simulink model "bat_cycling"  (R2021b)
settings: Solver=VariableStepAuto  StartTime=0.0  StopTime=3600*8640  RelTol=1e-3
undefined symbols (not defined in the file): Ion, Lithium
libraries: spsBatteryLib x1, spsControlledCurrentSourceLib x1, slpidlib x1, spspowerguiLib x1
settings Model: SimulationMode=accelerator  Creator=anna897  LastModifiedBy=anna897

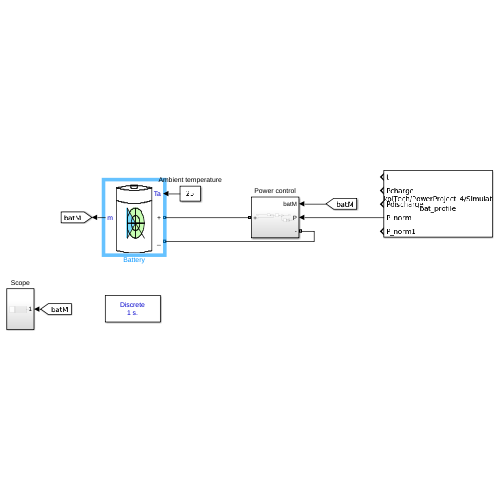
[thumbnail: Simulink's stored preview of the top-level diagram]
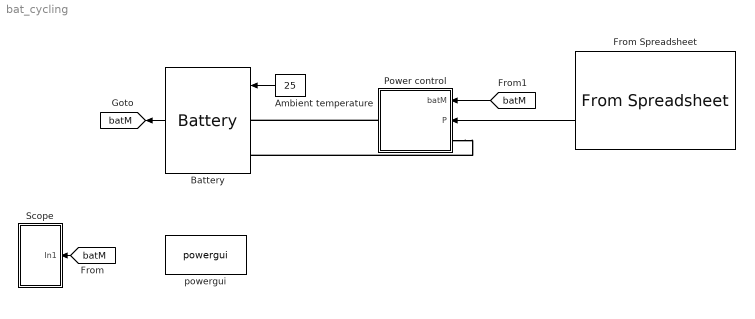
== system bat_cycling ==
  Ambient temperature : Constant  Value=25
  Battery : spsBatteryLib/Battery  BatType=Lithium-Ion  ShowTempParam=on  ThermalPreset=no  ShowAgeParam=on  NomV=7.2  NomQ=5.4  SOC=5  Batt_Tr=30  PresetModel=off  MaxQ=5.4  MinV=5.4  FullV=8.3807  Dis_rate=2.3478  R=0.3  Normal_OP=4.8835  expZone="[7.7788      0.2653]"  current=[6.5 13 32.5]  Units=Time  Tci=20  NomT=20  T2=-30  MaxQ2=4.8  FullV2=7.1  Normal_OP2=5.655  expZone2="[6.58           1]"  Rca=0.6  ti=2000  Dp=0  Neq0=0  Tsim=1  Ta1=25  Qeol=5.4*0.9  Reol=0.013333*1.2  Char_age=[2.3478, 3]  Dis_age=[2.3478, 10]  N1=1500  N2=10500  N3=1000  N4=1400  Ta2=45  N5=950
  From Spreadsheet : FromSpreadsheet  FileName=/home/anna897/SkolTech/PowerProject_4/Simulation/bat_profile.xls  SheetName=bat_profile  TreatFirstColumnAs=Data  SampleTime=3600
  Power control : Subsystem
  Scope : Subsystem
  powergui : spspowerguiLib/powergui  Priority=1  SimulationMode=Discrete  SampleTime=1  frequency=60  Iterations=50  frequencyindice=0  Pbase=100e6  ErrMax=1e-4  UnitsV=kV  UnitsW=MW  buscounter=0  FunctionMessages=off  echomessages=off  EnableUseOfTLC=off  CurrentSourceSwitches=off  DisableSnubberDevices=off  DisableRonSwitches=off  DisableVfSwitches=off  DisplayEquations=off  AutomaticDiscreteSolvers=off  SolverType=Tustin/Backward Euler (TBE)  Interpol=off  ExternalGateDelay=off  methode=off  Ts=100  x0status=blocks  SPID=on  SwTol=0  HookPort=off  NonlinearTolerance=1e-4  nMaxIteration=100  ContinueOnMaxIteration=off  RestoreLinks=warning  ResistiveCurrentMeasurement=off  Frange=[0:2:500]  Ylog=off  Xlog=on  ShowGrid=off  save=off  variable=ZData  structure=0  ZoomFFT=off  StartTime=0.0  cycles=1  DisplayStyle=1  fundamental=60  FreqAxis=off  MaxFrequency=1000  frequencyindicesteady=1  RmsSteady=1  display=off
  tag scope: batM=global
  wires:
  Ambient temperature/1 -> Battery/1
  Battery/1 -> [batM]
  [batM] -> Scope/1(In1)
  [batM] -> Power control/1(batM)
  From Spreadsheet/4 -> Power control/2(P)
  connections:
  Power control/RConn1 -- Battery/LConn1
  Power control/LConn1 -- Battery/LConn2

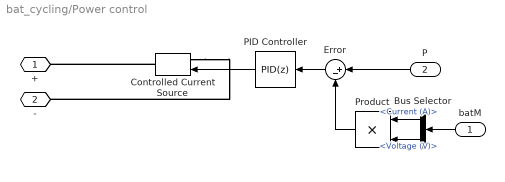
== system bat_cycling/Power control ==
  batM : Inport
  P : Inport  Port=2
  Bus Selector : BusSelector  OutputSignals=Current (A),Voltage (V)
  Controlled Current Source : spsControlledCurrentSourceLib/Controlled Current Source  Initialize=on  Source_Type=AC  Amplitude=0  Phase=0  Frequency=0  Measurements=None
  Error : Sum  Inputs=|+-
  PID Controller : slpidlib/PID Controller  Controller=PID  Form=Ideal  TimeDomain=Discrete-time  UseExternalTs=off  SampleTime=1  IntegratorMethod=Forward Euler  FilterMethod=Forward Euler  ControllerParametersSource=internal  P=1  I=0  D=0  UseFilter=off  N=100  TunerSelectOption=Transfer Function Based (PID Tuner App)  InitialConditionSource=internal  InitialConditionForIntegrator=0  InitialConditionForFilter=0  DifferentiatorICPrevScaledInput=0  ExternalReset=none  TrackingMode=off  Kt=1  LimitOutput=off  SatLimitsSource=internal  UpperSaturationLimit=inf  LowerSaturationLimit=-inf  LinearizeAsGain=on  AntiWindupMode=none  Kb=1  POutMin=[]  POutMax=[]  IOutMin=[]  IOutMax=[]  DOutMin=[]  DOutMax=[]  NOutMin=[]  NOutMax=[]  SumOutMin=[]  SumOutMax=[]  SaturationOutMin=[]  SaturationOutMax=[]  PParamMin=[]  PParamMax=[]  IParamMin=[]  IParamMax=[]  DParamMin=[]  DParamMax=[]  NParamMin=[]  NParamMax=[]  KbParamMin=[]  KbParamMax=[]  KtParamMin=[]  KtParamMax=[]  KbOutMin=[]  KbOutMax=[]  KtOutMin=[]  KtOutMax=[]  IntegratorOutMin=[]  IntegratorOutMax=[]  FilterOutMin=[]  FilterOutMax=[]  SumI1OutMin=[]  SumI1OutMax=[]  SumI2OutMin=[]  SumI2OutMax=[]  SumI3OutMin=[]  SumI3OutMax=[]  SumI4OutMin=[]  SumI4OutMax=[]  SumDOutMin=[]  SumDOutMax=[]  DifferentiatorOutMin=[]  DifferentiatorOutMax=[]  FilterDiffOutCoefMin=[]  FilterDiffOutCoefMax=[]  ReciprocalOutMin=[]  ReciprocalOutMax=[]  SumDenOutMin=[]  SumDenOutMax=[]  SumNumOutMin=[]  SumNumOutMax=[]  DivideOutMin=[]  DivideOutMax=[]  UdiffTsProdOutMin=[]  UdiffTsProdOutMax=[]  NTsProdOutMin=[]  NTsProdOutMax=[]  UintegralTsProdOutMin=[]  UintegralTsProdOutMax=[]  UngainTsProdOutMin=[]  UngainTsProdOutMax=[]  IntegratorContinuousStateAttributes=''  IntegratorStateMustResolveToSignalObject=off  IntegratorRTWStateStorageClass=Auto  FilterContinuousStateAttributes=''  FilterStateMustResolveToSignalObject=off  FilterRTWStateStorageClass=Auto  ParallelPVariant=Passthrough  IdealPVariant=InternalParameters  IVariant=InternalParameters  DVariant=InternalParameters  IntegratorVariant=Discrete  SatVariant=Disabled  AWVariant=Passthrough  PCopyVariant=Disabled  TRVariant=Disabled  FdbkBlocksVariant=Forward  IdealPFdbkVariant=Disabled  SatFdbkVariant=Disabled  DerivativeFilterVariant=Differentiator  NVariant=Passthrough  NCopyVariant=Disabled_SignalSpec  FilterICVariant=InternalICsDifferentiator  IntegratorICVariant=InternalICs  ExternalResetVariant=Disabled  TRSumVariant=Passthrough  SumFdbkVariant=Disabled  SumVariant=Sum_PID  TsampFilterVariant=InternalTs  TsampNgainVariant=Passthrough  TsampIntegralVariant=Passthrough  ExternalSaturationOutDataTypeStr=Inherit: Same as second input
  Product : Product
  + : PMIOPort  Side=Right
  - : PMIOPort  Port=2  Side=Left
  wires:
  PID Controller/1 -> Controlled Current Source/1
  Error/1 -> PID Controller/1
  P/1 -> Error/1
  batM/1 -> Bus Selector/1
  Product/1 -> Error/2
  Bus Selector/1 -> Product/1  "<Current (A)>"
  Bus Selector/2 -> Product/2  "<Voltage (V)>"
  connections:
  Controlled Current Source/RConn1 -- +/RConn1
  Controlled Current Source/LConn1 -- -/RConn1

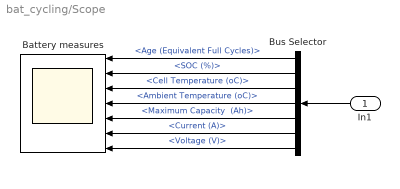
== system bat_cycling/Scope ==
  In1 : Inport
  Battery measures : Scope  NumInputPorts=7
  Bus Selector : BusSelector  OutputSignals="Age (Equivalent Full Cycles),SOC (%),Cell Temperature (oC),Ambient Temperature (oC),Maximum Capacity  (Ah),Current (A),Voltage (V)"
  wires:
  Bus Selector/1 -> Battery measures/1  "<Age (Equivalent Full Cycles)>"
  Bus Selector/5 -> Battery measures/5  "<Maximum Capacity  (Ah)>"
  Bus Selector/4 -> Battery measures/4  "<Ambient Temperature (oC)>"
  Bus Selector/7 -> Battery measures/7  "<Voltage (V)>"
  In1/1 -> Bus Selector/1
  Bus Selector/3 -> Battery measures/3  "<Cell Temperature (oC)>"
  Bus Selector/6 -> Battery measures/6  "<Current (A)>"
  Bus Selector/2 -> Battery measures/2  "<SOC (%)>"
